simulink model "UNICO"  (R2023b)
settings: Solver=FixedStepDiscrete  StartTime=0.0  StopTime=inf  FixedStep=Control.DT  RelTol=1e-3
undefined symbols (not defined in the file): Control
libraries: cstblocks x5, simulink x2
(part 2 of 3)

== system UNICO/Echo print/Enabled Subsystem ==
  Init : Inport
  Params : Inport  Port=2
  KpAr : Inport  Port=3
  KiAr : Inport  Port=4
  KpBr : Inport  Port=5
  KiBr : Inport  Port=6
  Max_Rat : Inport  Port=7
  Params_WS_F : Inport  Port=8
  Enable : EnablePort
  Echo1 : MATLAB Function  TreatAsAtomicUnit=on
  wires:
  Init/1 -> Echo1/1(Init)
  Params_WS_F/1 -> Echo1/8(Params_WS_F)
  Max_Rat/1 -> Echo1/7(Max_Rat)
  KiAr/1 -> Echo1/4(KiAr)
  KpAr/1 -> Echo1/3(KpAr)
  Params/1 -> Echo1/2(Params)
  KpBr/1 -> Echo1/5(KpBr)
  KiBr/1 -> Echo1/6(KiBr)

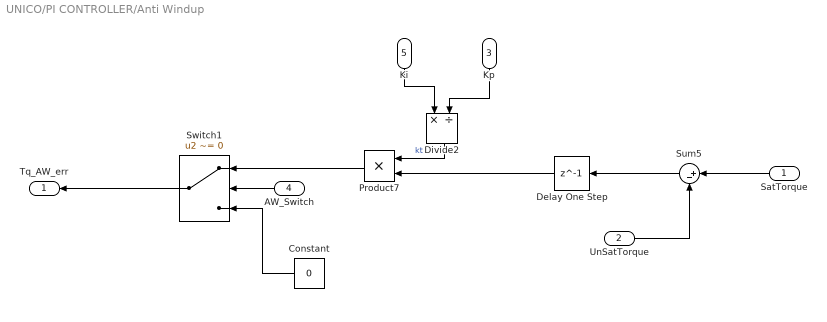
== system UNICO/PI CONTROLLER/Anti Windup ==
  SatTorque : Inport
  UnSatTorque : Inport  Port=2
  Kp : Inport  Port=3
  AW_Switch : Inport  Port=4
  Ki : Inport  Port=5
  Constant : Constant  Value=0
  Delay One Step : Delay  DelayLength=1
  Divide2 : Product  Inputs=*/
  Product7 : Product
  Sum5 : Sum  Inputs=|+-
  Switch1 : Switch  Criteria=u2 ~= 0  SaturateOnIntegerOverflow=off  InputSameDT=off
  Tq_AW_err : Outport
  wires:
  Sum5/1 -> Delay One Step/1
  Ki/1 -> Divide2/1
  SatTorque/1 -> Sum5/1
  Divide2/1 -> Product7/1  "kt"
  Delay One Step/1 -> Product7/2
  Kp/1 -> Divide2/2
  UnSatTorque/1 -> Sum5/2
  Product7/1 -> Switch1/1
  Switch1/1 -> Tq_AW_err/1
  Constant/1 -> Switch1/3
  AW_Switch/1 -> Switch1/2

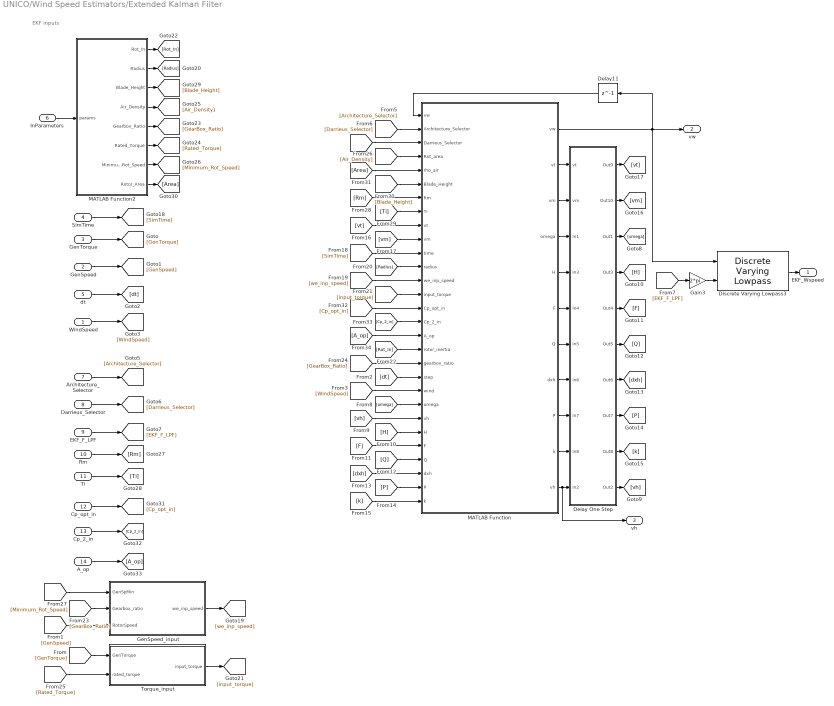
== system UNICO/Wind Speed Estimators/Extended Kalman Filter ==
  note: EKF inputs
  WindSpeed : Inport
  GenSpeed : Inport  Port=2
  GenTorque : Inport  Port=3
  SimTime : Inport  Port=4
  dt : Inport  Port=5
  InParameters : Inport  Port=6
  Architecture_Selector : Inport  Port=7
  Darrieus_Selector : Inport  Port=8
  EKF_F_LPF : Inport  Port=9
  Rm : Inport  Port=10
  Ti : Inport  Port=11
  Cp_opt_in : Inport  Port=12
  Cp_2_in : Inport  Port=13
  A_op : Inport  Port=14
  Delay One Step : Subsystem
  Delay11 : Delay  DelayLength=1
  Discrete Varying Lowpass3 : cstblocks/Linear Parameter Varying/Discrete Varying Lowpass  N=1  w0=0  Ts=Control.DT
  Gain3 : Gain  Gain=2*pi
  GenSpeed_input : MATLAB Function  TreatAsAtomicUnit=on
  MATLAB Function : MATLAB Function  TreatAsAtomicUnit=on
  MATLAB Function2 : MATLAB Function  TreatAsAtomicUnit=on
  Torque_input : MATLAB Function  TreatAsAtomicUnit=on
  EKF_Wspeed : Outport
  vw : Outport  Port=2
  vh : Outport  Port=3
  wires:
  [Radius] -> MATLAB Function/12(radius)
  [GearBox_Ratio] -> GenSpeed_input/2(Gearbox_ratio)
  [Minimum_Rot_Speed] -> GenSpeed_input/1(GenSpMin)
  [Rated_Torque] -> Torque_input/2(rated_torque)
  [Rot_In] -> MATLAB Function/18(rotor_inertia)
  Delay11/1 -> MATLAB Function/1("vw ")
  MATLAB Function/1(vw) -> vw/1, Delay11/1, Discrete Varying Lowpass3/1
  [EKF_F_LPF] -> Gain3/1
  Gain3/1 -> Discrete Varying Lowpass3/2
  Discrete Varying Lowpass3/1 -> EKF_Wspeed/1
  InParameters/1 -> MATLAB Function2/1(params)
  GenTorque/1 -> [GenTorque]
  [GenTorque] -> Torque_input/1(GenTorque)
  GenSpeed/1 -> [GenSpeed]
  [GenSpeed] -> GenSpeed_input/3(RotorSpeed)
  dt/1 -> [dt]
  [dt] -> MATLAB Function/20(step)
  WindSpeed/1 -> [WindSpeed]
  [WindSpeed] -> MATLAB Function/21(wind)
  Architecture_Selector/1 -> [Architecture_Selector]
  Darrieus_Selector/1 -> [Darrieus_Selector]
  EKF_F_LPF/1 -> [EKF_F_LPF]
  MATLAB Function/4(omega) -> Delay One Step/3(In1)
  MATLAB Function/5(H) -> Delay One Step/4(In3)
  MATLAB Function/6(F) -> Delay One Step/5(In4)
  MATLAB Function/7(Q) -> Delay One Step/6(In5)
  MATLAB Function/8(dxh) -> Delay One Step/7(In6)
  MATLAB Function/9(P) -> Delay One Step/8(In7)
  MATLAB Function/10(k) -> Delay One Step/9(In8)
  Delay One Step/3(Out1) -> [omega]
  Delay One Step/10(Out2) -> [vh]
  Delay One Step/4(Out3) -> [H]
  Delay One Step/5(Out4) -> [F]
  Delay One Step/6(Out5) -> [Q]
  Delay One Step/7(Out6) -> [dxh]
  Delay One Step/8(Out7) -> [P]
  Delay One Step/9(Out8) -> [k]
  [omega] -> MATLAB Function/22("omega ")
  [vh] -> MATLAB Function/23("vh ")
  [H] -> MATLAB Function/24("H ")
  [F] -> MATLAB Function/25("F ")
  [Q] -> MATLAB Function/26("Q ")
  [dxh] -> MATLAB Function/27("dxh ")
  [P] -> MATLAB Function/28("P ")
  [k] -> MATLAB Function/29("k ")
  MATLAB Function/3(vm) -> Delay One Step/2(vm)
  MATLAB Function/2(vt) -> Delay One Step/1(vt)
  Delay One Step/1(Out9) -> [vt]
  Delay One Step/2(Out10) -> [vm]
  [vt] -> MATLAB Function/9("vt ")
  [vm] -> MATLAB Function/10("vm ")
  SimTime/1 -> [SimTime]
  [SimTime] -> MATLAB Function/11(time)
  GenSpeed_input/1(we_inp_speed) -> [we_inp_speed]
  [we_inp_speed] -> MATLAB Function/13(we_inp_speed)
  MATLAB Function2/2(Radius) -> [Radius]
  Torque_input/1(input_torque) -> [input_torque]
  [input_torque] -> MATLAB Function/14(input_torque)
  MATLAB Function2/1(Rot_In) -> [Rot_In]
  MATLAB Function2/5(Gearbox_Ratio) -> [GearBox_Ratio]
  [GearBox_Ratio] -> MATLAB Function/19(gearbox_ratio)
  MATLAB Function2/6(Rated_Torque) -> [Rated_Torque]
  MATLAB Function2/4(Air_Density) -> [Air_Density]
  MATLAB Function2/7(Minimum_Rot_Speed) -> [Minimum_Rot_Speed]
  Rm/1 -> [Rm]
  Ti/1 -> [Ti]
  [Rm] -> MATLAB Function/7(Rm)
  [Ti] -> MATLAB Function/8(Ti)
  MATLAB Function2/3(Blade_Height) -> [Blade_Height]
  [Blade_Height] -> MATLAB Function/6(Blade_Height)
  [Air_Density] -> MATLAB Function/4(Rot_area)
  [Darrieus_Selector] -> MATLAB Function/3(Darrieus_Selector)
  [Architecture_Selector] -> MATLAB Function/2(Architecture_Selector)
  MATLAB Function2/8(Rotor_Area) -> [Area]
  [Area] -> MATLAB Function/5(rho_air)
  A_op/1 -> [A_op]
  Cp_2_in/1 -> [Cp_2_in]
  Cp_opt_in/1 -> [Cp_opt_in]
  [Cp_2_in] -> MATLAB Function/16(Cp_2_in)
  [Cp_opt_in] -> MATLAB Function/15(Cp_opt_in)
  [A_op] -> MATLAB Function/17(A_op)
  MATLAB Function/11(vh) -> vh/1, Delay One Step/10(In2)

== system UNICO/Wind Speed Estimators/Subsystem ==
  dt : Inport
  GenSpeed : Inport  Port=2
  Delay One Step : Delay  DelayLength=1
  Divide : Product  Inputs=*/
  Sum : Sum  Inputs=|+-
  GenAcc : Outport
  wires:
  GenSpeed/1 -> Sum/1, Delay One Step/1
  Delay One Step/1 -> Sum/2
  dt/1 -> Divide/2
  Sum/1 -> Divide/1
  Divide/1 -> GenAcc/1

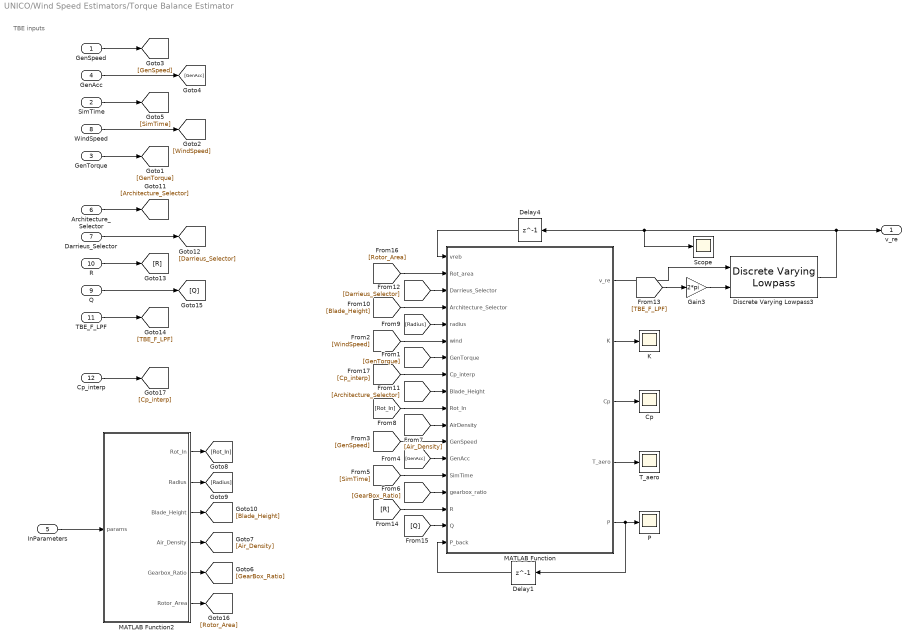
== system UNICO/Wind Speed Estimators/Torque Balance Estimator ==
  note: TBE inputs
  GenSpeed : Inport
  SimTime : Inport  Port=2
  GenTorque : Inport  Port=3
  GenAcc : Inport  Port=4
  InParameters : Inport  Port=5
  Architecture_Selector : Inport  Port=6
  Darrieus_Selector : Inport  Port=7
  WindSpeed : Inport  Port=8
  Q : Inport  Port=9
  R : Inport  Port=10
  TBE_F_LPF : Inport  Port=11
  Cp_interp : Inport  Port=12
  Cp : Scope
  Delay1 : Delay  DelayLength=1
  Delay4 : Delay  DelayLength=1
  Discrete Varying Lowpass3 : cstblocks/Linear Parameter Varying/Discrete Varying Lowpass  N=1  w0=0  Ts=Control.DT
  Gain3 : Gain  Gain=2*pi
  K : Scope
  MATLAB Function : MATLAB Function  TreatAsAtomicUnit=on
  MATLAB Function2 : MATLAB Function  TreatAsAtomicUnit=on
  P : Scope
  Scope : Scope
  T_aero : Scope
  v_re : Outport
  wires:
  Delay4/1 -> MATLAB Function/1(vreb)
  MATLAB Function/1(v_re) -> Discrete Varying Lowpass3/1
  [TBE_F_LPF] -> Gain3/1
  Gain3/1 -> Discrete Varying Lowpass3/2
  Discrete Varying Lowpass3/1 -> v_re/1, Delay4/1, Scope/1
  MATLAB Function/5(P) -> Delay1/1, P/1
  Delay1/1 -> MATLAB Function/18(P_back)
  MATLAB Function/2(K) -> K/1
  MATLAB Function/3(Cp) -> Cp/1
  MATLAB Function/4(T_aero) -> T_aero/1
  InParameters/1 -> MATLAB Function2/1(params)
  GenTorque/1 -> [GenTorque]
  [GenTorque] -> MATLAB Function/7(GenTorque)
  WindSpeed/1 -> [WindSpeed]
  [WindSpeed] -> MATLAB Function/6(wind)
  [GenSpeed] -> MATLAB Function/12(GenSpeed)
  GenSpeed/1 -> [GenSpeed]
  GenAcc/1 -> [GenAcc]
  [GenAcc] -> MATLAB Function/13(GenAcc)
  SimTime/1 -> [SimTime]
  [SimTime] -> MATLAB Function/14(SimTime)
  MATLAB Function2/5(Gearbox_Ratio) -> [GearBox_Ratio]
  [GearBox_Ratio] -> MATLAB Function/15(gearbox_ratio)
  [Air_Density] -> MATLAB Function/11(AirDensity)
  MATLAB Function2/4(Air_Density) -> [Air_Density]
  MATLAB Function2/1(Rot_In) -> [Rot_In]
  [Rot_In] -> MATLAB Function/10(Rot_In)
  MATLAB Function2/2(Radius) -> [Radius]
  MATLAB Function2/3(Blade_Height) -> [Blade_Height]
  [Blade_Height] -> MATLAB Function/4(Architecture_Selector)
  [Radius] -> MATLAB Function/5(radius)
  Architecture_Selector/1 -> [Architecture_Selector]
  [Architecture_Selector] -> MATLAB Function/9(Blade_Height)
  Darrieus_Selector/1 -> [Darrieus_Selector]
  [Darrieus_Selector] -> MATLAB Function/3(Darrieus_Selector)
  R/1 -> [R]
  Q/1 -> [Q]
  TBE_F_LPF/1 -> [TBE_F_LPF]
  [R] -> MATLAB Function/16(R)
  [Q] -> MATLAB Function/17(Q)
  MATLAB Function2/6(Rotor_Area) -> [Rotor_Area]
  [Rotor_Area] -> MATLAB Function/2(Rot_area)
  [Cp_interp] -> MATLAB Function/8(Cp_interp)
  Cp_interp/1 -> [Cp_interp]

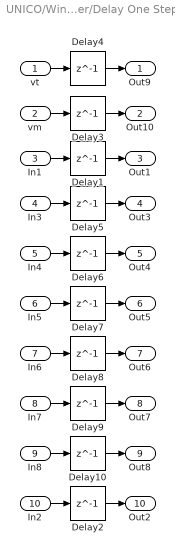
== system UNICO/Wind Speed Estimators/Extended Kalman Filter/Delay One Step ==
  vt : Inport
  vm : Inport  Port=2
  In1 : Inport  Port=3
  In3 : Inport  Port=4
  In4 : Inport  Port=5
  In5 : Inport  Port=6
  In6 : Inport  Port=7
  In7 : Inport  Port=8
  In8 : Inport  Port=9
  In2 : Inport  Port=10
  Delay{1..10} (10 alike) : Delay  DelayLength=1
  Out9 : Outport
  Out10 : Outport  Port=2
  Out1 : Outport  Port=3
  Out3 : Outport  Port=4
  Out4 : Outport  Port=5
  Out5 : Outport  Port=6
  Out6 : Outport  Port=7
  Out7 : Outport  Port=8
  Out8 : Outport  Port=9
  Out2 : Outport  Port=10
  wires:
  Delay8/1 -> Out6/1
  In7/1 -> Delay9/1
  Delay5/1 -> Out3/1
  Delay2/1 -> Out2/1
  In4/1 -> Delay6/1
  In1/1 -> Delay1/1
  In5/1 -> Delay7/1
  In6/1 -> Delay8/1
  In8/1 -> Delay10/1
  Delay9/1 -> Out7/1
  Delay6/1 -> Out4/1
  Delay7/1 -> Out5/1
  Delay10/1 -> Out8/1
  In2/1 -> Delay2/1
  In3/1 -> Delay5/1
  Delay1/1 -> Out1/1
  Delay4/1 -> Out9/1
  vt/1 -> Delay4/1
  vm/1 -> Delay3/1
  Delay3/1 -> Out10/1

== matlab function UNICO/PI CONTROLLER/Saturate  torque ==
  data: Unsat_Tq input; Gen_Tq output; Params input; time input
function Gen_Tq = fcn(Unsat_Tq, Params, time)


Min_Tq = Params(7);  %minimum torque value  [Nm]
Max_Tq = Params(8);  % maximum torque value  [Nm]

if time < -1   % at the beginning of the simulation do not apply torque saturation to avoid divergence
    Gen_Tq = Unsat_Tq;
else

    if Unsat_Tq > Max_Tq  % if torque from controller is larger than maximum saturation value
        

        Gen_Tq = Max_Tq;  % set the torque value to the MaxTq

    elseif Unsat_Tq < Min_Tq  % if torque from controller is smaller than minimum saturation value

        Gen_Tq = Min_Tq;  % set torque value to MinTq

    else   % if torque from controller is within the max and min values, do not modify the output torque value

        Gen_Tq = Unsat_Tq;


    end
end

== matlab function UNICO/Rate limiter ==
  data: Gen_Tq_b input; Gen_Tq input; s output; dMaxRate input; time input; dt input
function s = fcn(Gen_Tq_b,Gen_Tq,dMaxRate, time, dt)
% rate limiter applied only after *** seconds to allow for controller
% initialization
if time>0
    rate_lim_pos = dMaxRate; % rate limit for torque is simmetric
    rate_lim_neg = -dMaxRate;
    % calculate torque rate
    rate = (Gen_Tq-Gen_Tq_b)/dt;

    if rate > rate_lim_pos % if the torque rate is larger than the maximum allowed, set the torque using the maximum rate

        Gen_Tq = Gen_Tq_b+rate_lim_pos*dt;

    elseif rate < rate_lim_neg % if the torque rate is smaller than the minimum allowed, set the torque using the minimum rate

        Gen_Tq = Gen_Tq_b+rate_lim_neg*dt;

    end

else

end
% if the maximum torque rate is not violated
s = Gen_Tq;

== matlab function UNICO/MATLAB Function2 ==
  data: log1 input; y1 output; log2 input; log3 input; log4 input; y2 output; y3 output
function [y1, y2, y3] = log_to_file(log1, log2, log3, log4)
% log1      : [-]
% log2      : [-]
% log3      : [-]
% log4      : [-]

% y1, y2, y3 (pass-through)
y1 = log1;
y2 = log2;
y3 = log3;

persistent fid
if isempty(fid)
    % Corrected: used commas to separate arguments and removed extra semicolons
    fid = fopen('D:\Dario\Firenze_Maggio\Simulazioni_Sandia\UNICO_logger.txt', 'w');

    if fid == -1
        % Optional: use warning('Failed to open file'); to see if it fails in the console
        return;
    end

    % Standard header creation
    header = sprintf('log1[-]\tlog2[-]\tlog3[-]\tlog4[-]\n');
    fwrite(fid, header, 'char');
end

if fid ~= -1
    row = sprintf('%.6f\t%.6f\t%.6f\t%.6f\n', log1, log2, log3, log4);
    fwrite(fid, row, 'char');
end

== matlab function UNICO/Reference Speed Determination/WT_Controller ==
  data: WindSpeed input; GenSpeed input; GenSpeedRef output; Params input; Ref_Speed_F_Sw output; Ref_Speed_F_LPF output; Architecture_Selector input; Darrieus_Selector input
function [GenSpeedRef, Ref_Speed_F_Sw,Ref_Speed_F_LPF]  = WT_Controller(WindSpeed, GenSpeed, Params, Architecture_Selector, Darrieus_Selector)

% Load struct variables
R       = Params(1);                        % Rotor radius                                [m]
v_rt    = Params(2);                        % Rated wind speed                            [m/s]
Pt      = Params(4);                        % RatedPwr                                    [W]
w_rt    = Params(5);                        % RatedGenSpeed                               [rad/s]
eta     = Params(6);                        % Generator Efficiency                        [-]
w_min   = Params(9);                        % Minimum generator speed                     [rad/s]
r2      = Params(10);                       % Region 2 control mode                       [-]
TSR_opt = Params(15);                       % optimal TSR                                 [-]
Cpmaxval= Params(16);                       % max CP value                                [-]
r3      = Params(17);                       % Region 3 control mode                       [-]
m       = Params(18);                       % Angular coefficient Region 3 linear method  []
V_lin   = Params(19);                       % Wind speed to start linear reduction        [m/s]
TSR_R3 =  Params(26);                       % Region 3 Tip Speed Ratio                    [-]
Ref_Speed_F_Sw = Params(20);                % Reference speed filter switch               [-]
Ref_Speed_F_LPF = Params(21);               % Reference speed cut-off frequency           [Hz]
rho     = Params(22);                       % Air density                                 [kg/m^3]
Bld_Height = Params(24);                    %Blades Height (VAWT ONLY)                    [m]
Rot_area= Params(28);                       % Rotor Area (Eggbeater Type VAWT ONLY)       [m^2]

% Define parameters
v       = WindSpeed;                        % Reassign parameter
w_opt   = v*TSR_opt/R;                      % Optimum generator speed (corresponding to optimum TSR)
if Architecture_Selector == 2
    if Darrieus_Selector == 1
        A = Bld_Height*2*R;                 %Area for VAWT - H Type
    else
        A = Rot_area;                       %Area for VAWT - Eggbeater Type
    end
else
    A = pi*(R^2);                           %Area for HAWT
end

% Region 1 - Region 2 - Region 2 1/2
if v <= v_rt
    if r2 == 0
        w_ref = min(max(w_min,w_opt),w_rt);  
    else
        % for switching region
        if abs(w_rt-GenSpeed)<abs(w_min-GenSpeed)
            %region 2.5
            w_ref = w_rt;
        else
            % region 1.5
            w_ref = w_min;

        end

    end
       
% Region 3
else
    % Rated power tracking
    if r3 == 0
        Cp = Pt*eta/(0.5*rho*A*v^3);
        Cp    = min(max(0,Cp),Cpmaxval);
        TSR   = TSR_R3;
        w_ref = v*TSR/R;

    else %linear reduction 
        
        if v< V_lin
            w_ref = w_rt;
        else
            w_ref = w_rt+m*(v-V_lin);
            w_ref = max(w_ref,w_min);

        end
    end
end

GenSpeedRef = w_ref;  % PI controller reference rotational speed
end

== matlab function UNICO/Echo print/Enabled Subsystem/Echo1 ==
  data: Init input; Params input; KpAr input; KiAr input; KpBr input; KiBr input; Max_Rat input; Params_WS_F input
function fcn(Init, Params, KpAr, KiAr, KpBr, KiBr, Max_Rat, Params_WS_F)

R               = Params(1);  % Rotor radius [m]
v_rt            = Params(2);  % Rated wind speed  [m/s]
Rt_Tq           = Params(3);  % Rated torque  [Nm]
Pt              = Params(4);  % Rated Power [-]
w_rt            = Params(5);  % Rated Geerator Speed  [W]
eta             = Params(6);  % Generator Efficiency [-]
Min_Tq          = Params(7); % Minimum Torque [Nm]
Max_Tq          = Params(8);  % Maximum torque  [Nm]
w_min           = Params(9);  % Minimum generator speed  [rad/s]
r2              = Params(10);    % Region 2 control mode [-]
KSwitch         = Params(11);  % Switch for user defined k [-] 
Rgn2K           = Params(12);    %user defined K value [Nms^2/rad^2] 
SpdSwitch       = Params(13);  % velocity switch between Rgn 2 and 2 1/2 [rad/s]
w_minSwitch     = Params(14); % Velocity switch between Rgn 1.5 and 2 [rad/s]
TSR_opt         = Params(15);   %optimal TSR [-]
Cpmax           = Params(16);     % Optimal Cp [-]
r3              = Params(17);  % Region 3 control mode [-]
m               = Params(18);  % Angular coefficient Region 3 linear method
V_lin           = Params(19);  % Wind speed to start linear reduction [m/s]
Ref_Speed_F_Sw  = Params(20); % Reference speed filter switch [-]
Ref_Speed_F_LPF = Params(21); % Reference speed cut-off frequency [Hz]
rho             = Params(22);  % Air density             [kg/m^3]
Wind_Speed_F_Sw = Params_WS_F(1); % switch for wind speed Low-pass filter [-]
Wind_Speed_F_LPF= Params_WS_F(2); % wind speed low pass filter frequency [Hz]
Gen_Speed_F_Sw  = Params_WS_F(3); % Switch for generator speed low-pass filter [-]
Gen_Speed_F_LPF = Params_WS_F(4); % Generator speed low pass frequeny [Hz]




if Init == 0
    
f_echo = fopen('UNICO_echo.txt','w');
fprintf(f_echo,'UNICO CONTROLLER SIMULATION INPUT \n');
fprintf(f_echo,'Rotor radius [m]:                           %f \n',R);
fprintf(f_echo,'Rated wind speed [m/s]:                     %f \n',v_rt);
fprintf(f_echo,'Rated Torque [Nm]:                          %f \n',Rt_Tq);
fprintf(f_echo,'Rated power [W]:                            %f \n',Pt);
fprintf(f_echo,'Rated generator speed [rad/s]:              %f \n',w_rt);
fprintf(f_echo,'Generator efficiency [-]:                   %f \n',eta);
fprintf(f_echo,'Minimum Torque [Nm]:                        %f \n',Min_Tq);
fprintf(f_echo,'Maximum generator torque [Nm]:              %f \n',Max_Tq);
fprintf(f_echo,'Maximum generator torque rate [Nm/s]:       %f \n',Max_Rat);
fprintf(f_echo,'Minumum generator speed [rad/s]:            %f \n',w_min);
fprintf(f_echo, 'Region 2 control [-]:                      %f \n', r2);
fprintf(f_echo,'Switch for user defined K [-]:              %f \n',KSwitch);
fprintf(f_echo,'User defined K value [Nms^2/rad^2]:         %f \n',Rgn2K);
fprintf(f_echo,'Switch between Rgn2 and 2.5 [rad/s]:        %f \n',SpdSwitch);
fprintf(f_echo,'Switch between Rgn1.5 and 2 [rad/s]:        %f \n',w_minSwitch);
fprintf(f_echo,'Optimum TSR [-]:                            %f \n',TSR_opt);
fprintf(f_echo,'Maximum Cp value [-]:                       %f \n', Cpmax);
fprintf(f_echo,'Region 3 control [-]:                       %f \n',r3);
fprintf(f_echo,'Angular coefficient linear method []:       %f \n',m);
fprintf(f_echo,'Start reduction of ref velocity [m/s]:      %f \n', V_lin);
fprintf(f_echo,'Above rated PI Controller Kp [Nms/rad]:     %f \n',KpAr);
fprintf(f_echo,'Above rated PI Controller Ki [Nm/rad]:      %f \n',KiAr);
fprintf(f_echo,'Below rated PI Controller Kp [Nms/rad]:     %f \n',KpBr);
fprintf(f_echo,'Below rated PI Controller Ki [Nm/rad]:      %f \n',KiBr);
fprintf(f_echo,'Switch Wind speed filter [-]:               %f \n',Wind_Speed_F_Sw);
fprintf(f_echo,'Wind speed lowpass frequency[Hz]:           %f \n',Wind_Speed_F_LPF);
fprintf(f_echo,'Switch Generator speed filter [-]:          %f \n',Gen_Speed_F_Sw);
fprintf(f_echo,'Generator speed lowpass frequency [Hz]:     %f \n',Gen_Speed_F_LPF);
fprintf(f_echo,'Switch reference speed filter [-]:          %f \n',Ref_Speed_F_Sw);
fprintf(f_echo,'Reference speed lowpass frequency [Hz]:     %f \n',Ref_Speed_F_LPF);
fprintf(f_echo,'Air density [kg/m^3]:                       %f \n',rho);
fclose(f_echo);

end

== matlab function UNICO/Extract Signals & Filtering/MATLAB Function ==
  data: w0 input; freq input; Ts input; u input; y output
function y = discreteVaryingLowpass(w0, freq, Ts, u)
% DISCRETEVARYINGLOWPASS Implements a 1st-order variable Butterworth filter.
%
% INPUTS:
%   u    : Current input signal
%   freq : Cutoff frequency in rad/s (can vary at each step)
%   Ts   : Sample time in seconds
%   w0   : Pre-warping frequency (rad/s). Set to 0 for standard Tustin.
%
% OUTPUT:
%   y    : Filtered output signal

    % Persistent variables to maintain state between time steps
    persistent u_prev y_prev
    
    % Initialization on the first run
    if isempty(u_prev)
        u_prev = 0;
        y_prev = 0;
    end

    % --- 1. Pre-warping Gain (K) ---
    % Standard Bilinear (Tustin) transform uses K = 2/Ts.
    % If a pre-warping frequency w0 is provided, K is adjusted.
    if w0 <= 0
        K = 2 / Ts;
    else
        K = w0 / tan(w0 * Ts / 2);
    end

    % --- 2. Variable Coefficient Calculation ---
    % Continuous Transfer Function: H(s) = freq / (s + freq)
    % Substitution: s = K * (z-1) / (z+1)
    
    denominator = (K + freq);
    b0 = freq / denominator;
    b1 = b0;                     % For 1st order Tustin, b0 always equals b1
    a1 = (freq - K) / denominator;

    % --- 3. Difference Equation ---
    % Standard Direct Form I implementation:
    % y[n] = b0*u[n] + b1*u[n-1] - a1*y[n-1]
    y = b0*u + b1*u_prev - a1*y_prev;

    % --- 4. State Update ---
    u_prev = u;
    y_prev = y;
end

== matlab function UNICO/Pitch Controller/Saturate  pitch ==
  data: pitch_max input; u input; y output; pitch_min input
function y = fcn(pitch_max, u, pitch_min)

lim_sup = pitch_max;    % Maximum blade pitch angle value [rad]

lim_inf = pitch_min;    % Minimum blade pitch angle value [rad]

if u > lim_sup          % If balde pitch angle from controller is larger than maximum saturation value

    y = lim_sup;        % Set blade pitch angle value to the lim_sup

elseif u < lim_inf      % If blade picth angle from controller is smaller than minimum saturation value

    y = lim_inf;        % Set blade picth angle value to the lim_inf

else                    % If blade picth angle from controller is within the max and min values, do not modify the output blade picth angle value

    y = u;      

end

end

== matlab function UNICO/Notch Filter/MATLAB Function ==
  data: DesGenSpeed input; BladePassFreq output; InPar input
function BladePassFreq = calculateBladePassFreq(DesGenSpeed, InPar)

    N_blades = InPar(23);

    % Converts rad/s of the generator to Hz of blade passage
    BladePassFreq = (N_blades * DesGenSpeed) / (2 * pi);
    
end

== matlab function UNICO/Extract Signals & Filtering/MATLAB Function1 ==
  data: w0 input; freq input; Ts input; u input; y output
function y = discreteVaryingLowpass(w0, freq, Ts, u)
% DISCRETEVARYINGLOWPASS Implements a 1st-order variable Butterworth filter.
%
% INPUTS:
%   u    : Current input signal
%   freq : Cutoff frequency in rad/s (can vary at each step)
%   Ts   : Sample time in seconds
%   w0   : Pre-warping frequency (rad/s). Set to 0 for standard Tustin.
%
% OUTPUT:
%   y    : Filtered output signal

    % Persistent variables to maintain state between time steps
    persistent u_prev y_prev
    
    % Initialization on the first run
    if isempty(u_prev)
        u_prev = 0;
        y_prev = 0;
    end

    % --- 1. Pre-warping Gain (K) ---
    % Standard Bilinear (Tustin) transform uses K = 2/Ts.
    % If a pre-warping frequency w0 is provided, K is adjusted.
    if w0 <= 0
        K = 2 / Ts;
    else
        K = w0 / tan(w0 * Ts / 2);
    end

    % --- 2. Variable Coefficient Calculation ---
    % Continuous Transfer Function: H(s) = freq / (s + freq)
    % Substitution: s = K * (z-1) / (z+1)
    
    denominator = (K + freq);
    b0 = freq / denominator;
    b1 = b0;                     % For 1st order Tustin, b0 always equals b1
    a1 = (freq - K) / denominator;

    % --- 3. Difference Equation ---
    % Standard Direct Form I implementation:
    % y[n] = b0*u[n] + b1*u[n-1] - a1*y[n-1]
    y = b0*u + b1*u_prev - a1*y_prev;

    % --- 4. State Update ---
    u_prev = u;
    y_prev = y;
end

== matlab function UNICO/Region Switch  ==
  data: WindSpeed input; GenSpeed input; PI_GenTq input; Architecture_Selector input; Darrieus_Selector input; GenTq output; Params input
function GenTq = Rgn2_Fcn(WindSpeed, GenSpeed, PI_GenTq, Architecture_Selector, Darrieus_Selector, Params)

% Load R struct variables
R       = Params(1);                        % Rotor radius                              [m]
v_rt    = Params(2);                        % Rated power wind speed                    [m/s]
w_rt    = Params(5);                        % Rated generator speed                     [rad/s]
w_min   = Params(9);                        % Minimum generator speed                   [rad/s]
r2      = Params(10);                       % Region 2 control mode  {0: optimum tsr tracking; 1: kw^2 torque law}
KSwitch = Params(11);                       % switch for user defined k
Rgn2K = Params(12);                         % user defined k {used only if KSwitch = 1}
SpdSwitch = Params(13);                     % speed switch from region 2 to 2 2 1/2     [rad/s]
w_minSwitch = Params(14);                   % Switch between region 1.5 and 2           [rad/s]
TSR_opt = Params(15);                       % Optimum TSR                               [-]
Cpmax = Params(16);                         % max cp value                              [-]
rho     = Params(22);                       % Air density                               [kg/m^3]
Bld_Height = Params(24);                    % Blades Height (VAWT ONLY)                 [m]            
Rot_area = Params(28);                      %Rotor Area (VAWT - Eggbeater Type ONLY)    [m^2]

% Define parameters
wg  = GenSpeed;
v   = WindSpeed;
if KSwitch == 1
    K = Rgn2K;
else
    if Architecture_Selector == 1
        K   = 0.5*rho*pi*R^5*Cpmax/TSR_opt^3;  % K coefficient for HAWT
    else
        if Darrieus_Selector == 1
             K   = rho*R^4*Bld_Height*Cpmax/TSR_opt^3;  % K coefficient for VAWT - H Type
        else
             K = 0.5*rho*Rot_area*R^3*Cpmax/TSR_opt^3;  % K coefficient for VAWT - Eggbeater Type
        end
    end
end
w1  = SpdSwitch;            % switching rotational speed for region 2.5 to 3
Tg1 = K*w1^2;               % torque value at the switching rotational speed
w2 = w_minSwitch;           % switching rotational speed for region 1.5 to 2
Tg2 = K*(w2)^2;             % generator torque at the switching rotational speed from k-w^2 law
Tgmin = K*w_min^2;          % generator torque at minimum rotational speed from k-w^2 law

% kw^2 control mode
if r2 == 1

    % if we are in region 1.5 or 2
    if (wg < w1) && (v <= v_rt)
        % use k-w^2 law
        GenTq =  K*wg^2;
        if wg < w2 % if the generator speed is smaller than the 1.5 switching value
            if PI_GenTq < Tg2 && PI_GenTq > Tgmin

                % use linear interpolation to smooth the switch between the two
                % regions
                GenTq = Tg2+(PI_GenTq-Tg2)/(w_min-w2)*(wg-w2);
               
            elseif PI_GenTq < Tgmin

                % in region 1.5 use TSR tracking to track the minimum speed
                % defined by the user
                GenTq = PI_GenTq;
                
            end
        end

    elseif (wg < w_rt) && (v <= v_rt)
        % region 2.5, smoothing of switch between region 2 and 3
        GenTq = Tg1+(PI_GenTq-Tg1)/(w_rt-w1)*(wg-w1);
    else
        % region 3
        GenTq = PI_GenTq;
    end
    % tsr tracking control mode
else
    GenTq = PI_GenTq;
end

== matlab function UNICO/Set Point Smoother/Rated_Power ==
  data: params input; y output
function y = fcn(params)
% extracting Turbine rated power from In_Parameters vector
y = params(4);  % Rated Power [W]

end

== matlab function UNICO/Set Point Smoother/MATLAB Function ==
  data: params input; w_rt output
function w_rt = fcn(params)
% extracting the reference generator speed  
w_rt = params(5);  

end

== matlab function UNICO/Extract Signals & Filtering/MATLAB Function2 ==
  data: w0 input; freq input; Ts input; u input; y output
function y = discreteVaryingLowpass(w0, freq, Ts, u)
% DISCRETEVARYINGLOWPASS Implements a 1st-order variable Butterworth filter.
%
% INPUTS:
%   u    : Current input signal
%   freq : Cutoff frequency in rad/s (can vary at each step)
%   Ts   : Sample time in seconds
%   w0   : Pre-warping frequency (rad/s). Set to 0 for standard Tustin.
%
% OUTPUT:
%   y    : Filtered output signal

    % Persistent variables to maintain state between time steps
    persistent u_prev y_prev
    
    % Initialization on the first run
    if isempty(u_prev)
        u_prev = 0;
        y_prev = 0;
    end

    % --- 1. Pre-warping Gain (K) ---
    % Standard Bilinear (Tustin) transform uses K = 2/Ts.
    % If a pre-warping frequency w0 is provided, K is adjusted.
    if w0 <= 0
        K = 2 / Ts;
    else
        K = w0 / tan(w0 * Ts / 2);
    end

    % --- 2. Variable Coefficient Calculation ---
    % Continuous Transfer Function: H(s) = freq / (s + freq)
    % Substitution: s = K * (z-1) / (z+1)
    
    denominator = (K + freq);
    b0 = freq / denominator;
    b1 = b0;                     % For 1st order Tustin, b0 always equals b1
    a1 = (freq - K) / denominator;

    % --- 3. Difference Equation ---
    % Standard Direct Form I implementation:
    % y[n] = b0*u[n] + b1*u[n-1] - a1*y[n-1]
    y = b0*u + b1*u_prev - a1*y_prev;

    % --- 4. State Update ---
    u_prev = u;
    y_prev = y;
end

== matlab function UNICO/Wind Speed Estimators/Torque Balance Estimator/MATLAB Function ==
  data: vreb input; Rot_area input; Darrieus_Selector input; Architecture_Selector input; radius input; wind input; GenTorque input; Cp_interp input; Blade_Height input; v_re output; K output; Cp output; T_aero output; Rot_In input; AirDensity input; GenSpeed input; GenAcc input; SimTime input; gearbox_ratio input; R input; Q input; P_back input; P output
function [v_re,K,Cp,T_aero,P] = fcn(vreb,Rot_area, Darrieus_Selector, Architecture_Selector, radius,wind,GenTorque,Cp_interp, Blade_Height, Rot_In,AirDensity,GenSpeed,GenAcc,SimTime,gearbox_ratio,R, Q, P_back)
if Architecture_Selector == 2
    if Darrieus_Selector == 1
        A = Blade_Height*2*radius; % Area VAWT - H Type
    else
        A = Rot_area; % Area VAWT - Eggbeater Type
    end
else
    A=pi*(radius)^2; % Area HAWT
end

% Initialization
if SimTime < 6 % If time is less than 6 seconds, set initial values
    v_re=wind;    % Set estimated wind speed equal to actual wind speed
    P=1;          % Initialize state estimation error covariance
    K=0;          % Initialize Kalman gain factor
    Cp=0;         % Initialize power coefficient
    T_aero=0;     % Initialize aerodynamic torque
else
    Cp=Cp_interp;                                           % Cp already interpolated in C
    Tfriction=0.04*GenTorque;                               % Calculate friction torque
    Trotor=Rot_In*GenAcc;                                   % Calculate rotor torque from inertia
    T_aero=Trotor+GenTorque*gearbox_ratio+Tfriction;        % Compute aerodynamic torque from torque balance
    vre_cub=T_aero*2*GenSpeed/(AirDensity*A*Cp);            % Compute the cube of the estimated effective wind speed
    vre=nthroot(vre_cub,3);                                 % Compute the effective wind speed
    P_pred=P_back+Q;                                        % Compute state estimation error covariance from the previous step
    y=vre-vreb;                                             % Compute the wind speed difference between the predicted and the value from the previous step
    K=P_pred/(P_pred+R);                                    % Compute Kalman gain factor
    v_re=vreb+K*y;                                          % Update estimated wind speed
    P=(1-K)*P_pred;                                         % Update state estimation error covariance
end
end

== matlab function UNICO/Extract Signals & Filtering/MATLAB Function3 ==
  data: w0 input; freq input; Ts input; u input; y output
function y = discreteVaryingLowpass(w0, freq, Ts, u)
% DISCRETEVARYINGLOWPASS Implements a 1st-order variable Butterworth filter.
%
% INPUTS:
%   u    : Current input signal
%   freq : Cutoff frequency in rad/s (can vary at each step)
%   Ts   : Sample time in seconds
%   w0   : Pre-warping frequency (rad/s). Set to 0 for standard Tustin.
%
% OUTPUT:
%   y    : Filtered output signal

    % Persistent variables to maintain state between time steps
    persistent u_prev y_prev
    
    % Initialization on the first run
    if isempty(u_prev)
        u_prev = 0;
        y_prev = 0;
    end

    % --- 1. Pre-warping Gain (K) ---
    % Standard Bilinear (Tustin) transform uses K = 2/Ts.
    % If a pre-warping frequency w0 is provided, K is adjusted.
    if w0 <= 0
        K = 2 / Ts;
    else
        K = w0 / tan(w0 * Ts / 2);
    end

    % --- 2. Variable Coefficient Calculation ---
    % Continuous Transfer Function: H(s) = freq / (s + freq)
    % Substitution: s = K * (z-1) / (z+1)
    
    denominator = (K + freq);
    b0 = freq / denominator;
    b1 = b0;                     % For 1st order Tustin, b0 always equals b1
    a1 = (freq - K) / denominator;

    % --- 3. Difference Equation ---
    % Standard Direct Form I implementation:
    % y[n] = b0*u[n] + b1*u[n-1] - a1*y[n-1]
    y = b0*u + b1*u_prev - a1*y_prev;

    % --- 4. State Update ---
    u_prev = u;
    y_prev = y;
end

== matlab function UNICO/Extract Signals & Filtering/MATLAB Function4 ==
  data: w0 input; freq input; Ts input; u input; y output
function y = discreteVaryingLowpass(w0, freq, Ts, u)
% DISCRETEVARYINGLOWPASS Implements a 1st-order variable Butterworth filter.
%
% INPUTS:
%   u    : Current input signal
%   freq : Cutoff frequency in rad/s (can vary at each step)
%   Ts   : Sample time in seconds
%   w0   : Pre-warping frequency (rad/s). Set to 0 for standard Tustin.
%
% OUTPUT:
%   y    : Filtered output signal

    % Persistent variables to maintain state between time steps
    persistent u_prev y_prev
    
    % Initialization on the first run
    if isempty(u_prev)
        u_prev = 0;
        y_prev = 0;
    end

    % --- 1. Pre-warping Gain (K) ---
    % Standard Bilinear (Tustin) transform uses K = 2/Ts.
    % If a pre-warping frequency w0 is provided, K is adjusted.
    if w0 <= 0
        K = 2 / Ts;
    else
        K = w0 / tan(w0 * Ts / 2);
    end

    % --- 2. Variable Coefficient Calculation ---
    % Continuous Transfer Function: H(s) = freq / (s + freq)
    % Substitution: s = K * (z-1) / (z+1)
    
    denominator = (K + freq);
    b0 = freq / denominator;
    b1 = b0;                     % For 1st order Tustin, b0 always equals b1
    a1 = (freq - K) / denominator;

    % --- 3. Difference Equation ---
    % Standard Direct Form I implementation:
    % y[n] = b0*u[n] + b1*u[n-1] - a1*y[n-1]
    y = b0*u + b1*u_prev - a1*y_prev;

    % --- 4. State Update ---
    u_prev = u;
    y_prev = y;
end

== matlab function UNICO/Wind Speed Estimators/Extended Kalman Filter/MATLAB Function ==
  data: vw input; Architecture_Selector input; Darrieus_Selector input; Rot_area input; rho_air input; Blade_Height input; Rm input; Ti input; vw output; vt input; vm input; time input; vt output; radius input; we_inp_speed input; input_torque input; vm output; omega output; H output size=[1 3]; F output size=[3 3]; Q output size=[3 3]; dxh output size=[3 1]; P output size=[3 3]; k output size=[3 1]; vh output; Cp_opt_in input; Cp_2_in input; A_op input; rotor_inertia input; gearbox_ratio input; step input; wind input; omega input; vh input; H input size=[1 3]; F input size=[3 3]; Q input size=[3 3]; dxh input size=[3 1]; P input size=[3 3]; k input size=[3 1]
function [vw,vt,vm,omega,H,F,Q,dxh,P,k,vh] = fcn(vw,Architecture_Selector, Darrieus_Selector, Rot_area, rho_air, Blade_Height, Rm, Ti, vt,vm,time,radius,we_inp_speed,input_torque,Cp_opt_in,Cp_2_in,A_op,rotor_inertia,gearbox_ratio,step,wind,omega,vh,H,F,Q,dxh,P,k)
L=6*radius; % Define the turbulence length scale
I=eye(3);
% Initialization
if time < 10
    omega=we_inp_speed;             % Set initial rotor speed
    vt=0;                           % Initialize turbulence-induced wind speed
    vm=wind;                        % Set initial mean wind speed
    vh=wind;                        % Set initial hub-height wind speed
    H=[1,0,0];                      % Measurement matrix
    F=zeros(3,3);                   % Initialize system dynamics matrix
    Q=zeros(3,3);                   % Initialize process noise covariance matrix
    dxh=zeros(3,1);                 % Initialize state derivative vector
    P=[0.01,0,0;0,0.01,0;0,0,1];    % Initialize state covariance matrix
    k=zeros(3,1);                   % Initialize Kalman gain
    vw=vt+vm;                       % Compute total wind speed
% Extended Kalman Filter (EKF) based on Abbas' approach
else
    % Update state vector with current values
    xh=[omega;vt;vm];
    dt=step;            % Time step size

    if Architecture_Selector == 2
        if Darrieus_Selector == 1
            Area = Blade_Height*2*radius;
        else
            Area = Rot_area;
        end
    else
        Area=pi*(radius^2);           % Rotor swept area
    end

    % Cp_opt and Cp_2 already interpolated in C using vh and vw
    Cp_opt = Cp_opt_in;
    Cp_2 = Cp_2_in;

    % Define system dynamics matrix F (A_op already interpolated in C)
    F(1,1)=A_op;
    F(1,2)=rho_air*Area*3*Cp_opt*(vh^2)/(omega*2*rotor_inertia);
    F(1,3)=F(1,2);
    F(2,2)=-pi*vm/(2*L);
    F(2,3)=-pi*vt/(2*L);

    % Define process noise covariance matrix Q
    Q(1,1)=0.00001;
    Q(2,2)=pi*(vm^3)*(Ti^2)/L;
    Q(3,3)=4/600;

    % Compute additional system parameters
    a=pi*vm/(2*L);

    % Compute aerodynamic torque
    tau=0.5*rho_air*Area*(vw^3)*Cp_2/we_inp_speed;

    % Compute state derivatives
    dxh(1,1)=(tau-gearbox_ratio*input_torque)/rotor_inertia;
    dxh(2,1)=-a*vt;
    dxh(3,1)=0;

    % Update state vector
    xh=xh+dxh*dt;

    % Update state covariance matrix
    P=P+dt*(F*P+P*F'+Q-k*Rm*k');

    % Compute Kalman gain
    S=(H*(P*H'))+Rm;
    k=P*H'/S;

    % Correct state estimate using Kalman filter
    xh=xh+k*(we_inp_speed-omega);
    P=(I-k*H)*P;

    % Extract updated state values
    omega=xh(1,1);      % Rotor speed
    vt=xh(2,1);         % Turbulence-induced wind speed
    vm=xh(3,1);         % Mean wind speed
    vh=vt+vm;           % Hub-height wind speed
    vw=vm+vt;           % Estimated (total) wind speed
end
end

== matlab function UNICO/Set Point Smoother/Gen_Ref_Pitch ==
  data: params input; delta_omega input; y output
function y = fcn(params, delta_omega)
% defining the new generator speed reference for the pitch controller
w_rt = params(5);  %Rated Generetor Speed as a Reference for pitch Control [rad/s]
 
if delta_omega < 0                  % In Region 2.5 modify the reference generator speed to avoid conflict with pitch controller

    y = w_rt - delta_omega;         % Following Abbas's rules

else                                % In Region 3 do no modify the reference generator speed

    y = w_rt;

end

end

== matlab function UNICO/Wind Speed Estimators/Extended Kalman Filter/GenSpeed_input ==
  data: GenSpMin input; we_inp_speed output; Gearbox_ratio input; RotorSpeed input
function we_inp_speed = fcn(GenSpMin,Gearbox_ratio,RotorSpeed)
% Function to ensure the rotor speed does not fall below a minimum threshold

if RotorSpeed < 0.25*GenSpMin/Gearbox_ratio         % Check if the rotor speed is below 25% of the minimum generator speed, adjusted by the gearbox ratio
    
    we_inp_speed = 0.25*GenSpMin/Gearbox_ratio;     % Set the input speed to the minimum allowable value

else                                                % Otherwise, use the actual rotor speed

    we_inp_speed = RotorSpeed;

end

end

== matlab function UNICO/Pitch Rate Limiter/Rate limiter ==
  data: u_b input; u input; s output; Pitch_Rate input; dt input
function s = fcn(u_b,u,Pitch_Rate, dt)

rate_lim_pos = Pitch_Rate; % rate limit for pitch is simmetric
rate_lim_neg = -Pitch_Rate;

% calculate pitch rate
rate = (u-u_b)/dt;

if rate > rate_lim_pos % if the pitch rate is larger than the maximum allowed, set the pitch using the maximum rate

    s = u_b+rate_lim_pos*dt;

elseif rate < rate_lim_neg % if the pitch rate is smaller than the minimum allowed, set the pitch using the minimum rate

    s = u_b+rate_lim_neg*dt;

else

    s = u;  % if the maximum pitch rate is not violated

end

== matlab function UNICO/Wind Speed Estimators/Extended Kalman Filter/Torque_input ==
  data: GenTorque input; input_torque output; rated_torque input
function input_torque = fcn(GenTorque,rated_torque)
% Function to limit the generator torque to a minimum threshold

if GenTorque < 0.001*rated_torque               % If the generator torque is below 0.001 times the rated torque
    
    input_torque = 0.001*rated_torque;          % Set the input torque to the minimum allowable value

else                                            % Otherwise, use the actual generator torque

    input_torque = GenTorque;

end

end

== matlab function UNICO/Wind Speed Estimators/MATLAB Function ==
  data: WSE_Mode input; TBE_WSpeed input; Raw_WSpeed input; WSpeed output; EKF_WSpeed input
function WSpeed = fcn(WSE_Mode, TBE_WSpeed, Raw_WSpeed, EKF_WSpeed)
if WSE_Mode == 1
    WSpeed = TBE_WSpeed;
elseif WSE_Mode == 2
    WSpeed = EKF_WSpeed;
else
    WSpeed = Raw_WSpeed;
end

== matlab function UNICO/Set Point Smoother/GenSpeed_Ref_Torque_Controller ==
  data: Gen_Ref_torq input; delta_omega input; y output
function y = fcn(Gen_Ref_torq, delta_omega)
% Defining the new generator speed reference for the torque controller

if delta_omega >= 0                     % In Region 2.5 and 3 modify the reference generator speed to avoid conflict with pitch controller

    y = Gen_Ref_torq - delta_omega;     % Following Abbas's rules

else                                    % In Region 2 do no modify the reference generator speed

    y = Gen_Ref_torq;                   

end

end

== matlab function UNICO/Wind Speed Estimators/Extended Kalman Filter/MATLAB Function2 ==
  data: params input; Rot_In output; Radius output; Blade_Height output; Air_Density output; Gearbox_Ratio output; Rated_Torque output; Minimum_Rot_Speed output; Rotor_Area output
function [Rot_In, Radius, Blade_Height, Air_Density, Gearbox_Ratio, Rated_Torque, Minimum_Rot_Speed, Rotor_Area] = fcn(params)
% extracting the generator speed reference   
Radius = params(1); 
Air_Density = params(22);
Blade_Height = params(24);
Rot_In = params(25);
Gearbox_Ratio = params(27);
Rotor_Area = params(28);
Rated_Torque = params(3);
Minimum_Rot_Speed = params(9);
end

== matlab function UNICO/Extract Signals & Filtering/Filtering Block  ==
  data: windNF input; wnd output; wind input; GenSpeedNF input; GenSpeed input; Pitch input; PitchNF input; Tq input; TqNF input; Pwr input; PwrNF input; time input; omega output; ptch output; torque output; Power output; LPF_Starting_Time input
function [wnd,omega,ptch,torque,Power] = fcn(windNF, wind,GenSpeedNF, GenSpeed, Pitch, PitchNF, Tq, TqNF, Pwr, PwrNF, time, LPF_Starting_Time)

% At the beginning of the simulation do not apply filtering to avoid divergence

if time > LPF_Starting_Time

    wnd=wind;        % Wind speed filtered

    omega=GenSpeed;  % Generator speed filtered

    ptch=Pitch;      % Blade picth angle filtered

    torque=Tq;       % Generator torque filtered

    Power=Pwr;       % Generator power filtered

else

    wnd=windNF;         % Wind speed unfiltered

    omega=GenSpeedNF;   % Generator speed unfiltered

    ptch=PitchNF;       % Blade picth angle unfiltered

    torque=TqNF;        % Generator torque unfiltered

    Power=PwrNF;        % Generator power unfiltered

end

== matlab function UNICO/Wind Speed Estimators/Torque Balance Estimator/MATLAB Function2 ==
  data: params input; Rot_In output; Radius output; Blade_Height output; Air_Density output; Gearbox_Ratio output; Rotor_Area output
function [Rot_In, Radius, Blade_Height, Air_Density, Gearbox_Ratio, Rotor_Area]    = fcn(params)
% extracting the generator speed reference 
Radius = params(1); 
Rot_In = params(25);
Blade_Height = params(24);
Air_Density = params(22);
Gearbox_Ratio = params(27);
Rotor_Area = params(28);

end

== matlab function UNICO/Notch Filter/MATLAB Function2 ==
  data: SimTime input; GenSpeedUnfiltered input; GenSpeedFiltered input; Genspeed output
function Genspeed = fcn(SimTime, GenSpeedUnfiltered, GenSpeedFiltered)
Transient = 0;
if SimTime > Transient
Genspeed = GenSpeedFiltered ;
else 
Genspeed =  GenSpeedUnfiltered;
end

== matlab function UNICO/Notch Filter/MATLAB Function3 ==
  data: u input; Ts input; f0 input; Filt_GenTq output; zeta_z input; zeta_p input
function Filt_GenTq = notch_filter(u, Ts, f0, zeta_z, zeta_p)

persistent x1 x2 y1 y2 last_f0 last_Ts last_zz last_zp ...
           b0 b1 b2 a1 a2

% Initialize on first run
if isempty(x1)
    x1 = 0; x2 = 0;
    y1 = 0; y2 = 0;

    last_f0 = -1;
    last_Ts = -1;
    last_zz = -1;
    last_zp = -1;

    b0 = 1; b1 = 0; b2 = 0;
    a1 = 0; a2 = 0;
end

% Recompute coefficients only when parameters change AND Ts > 0
if (f0 ~= last_f0) || (Ts ~= last_Ts) || ...
   (zeta_z ~= last_zz) || (zeta_p ~= last_zp)

    if Ts > 0
        omega0 = 2*pi*f0;
        K  = 2 / Ts;
        K2 = K * K;
        w2 = omega0 * omega0;

        % Bilinear (Tustin) transform — numerator
        bz0 = K2 + 2*zeta_z*omega0*K + w2;
        bz1 = 2*w2 - 2*K2;
        bz2 = K2 - 2*zeta_z*omega0*K + w2;

        % Bilinear (Tustin) transform — denominator
        az0 = K2 + 2*zeta_p*omega0*K + w2;
        az1 = 2*w2 - 2*K2;
        az2 = K2 - 2*zeta_p*omega0*K + w2;

        % Normalize so a[0] = 1
        b0 = bz0 / az0;
        b1 = bz1 / az0;
        b2 = bz2 / az0;
        a1 = az1 / az0;
        a2 = az2 / az0;
    end
    % Always cache the current parameters (even when Ts=0)
    % so the next call (Ts=dt>0) recomputes correctly
    last_f0 = f0;
    last_Ts = Ts;
    last_zz = zeta_z;
    last_zp = zeta_p;
end

% IIR difference equation
Filt_GenTq = b0*u + b1*x1 + b2*x2 - a1*y1 - a2*y2;

% Update delay states
x2 = x1;
x1 = u;
y2 = y1;
y1 = Filt_GenTq;

end

== matlab function UNICO/PI CONTROLLER/Gain scheduling ==
  data: GenSpeed input; WindSpeed input; kp_ar input; Ki output; ki_ar input; kp_br input; ki_br input; Kp output; Params input
function [Ki,Kp] = fcn(GenSpeed, WindSpeed, kp_ar, ki_ar,kp_br, ki_br, Params)

R       = Params(1);  % Rotor radius           [m]
v_rt    = Params(2);  % Rated power wind speed [m/s]
w_rt    = Params(5);  % Rated generator speed  [rad/s]
r2      = Params(10);  % Region 2 control mode  {0: optimum tsr tracking; 1: kw^2 torque law}
SpdSwitch = Params(13); %generator speed for switch between region 2 and 2 1/2

% if we use TSR tracking in below rated conditions, schedule the PI
% coefficients
if r2 == 0

    if WindSpeed < v_rt && GenSpeed < w_rt

        % if GenSpeed <=SpdSwitch
        if GenSpeed <= SpdSwitch
            Kp = kp_br;
            Ki = ki_br;

        elseif GenSpeed > SpdSwitch && GenSpeed <w_rt
            % else

            Kp = kp_br+(kp_ar-kp_br)/(w_rt-SpdSwitch)*(GenSpeed-SpdSwitch);
            Ki = ki_br+(ki_ar-ki_br)/(w_rt-SpdSwitch)*(GenSpeed-SpdSwitch);

        else

            Kp = kp_ar;
            Ki = ki_ar;
            % end
        end


    else

        Kp = kp_ar;
        Ki = ki_ar;
    end

else
    % if k-w is used only a set of kp and ki is used
    Kp = kp_ar;
    Ki = ki_ar;

end

== matlab function UNICO/MATLAB Function1 ==
  data: dFPitch input; Pitch_Controller_Out input; Pitch_out output
function Pitch_out = Pitch_Switch(dFPitch, Pitch_Controller_Out)

if dFPitch <= -99
    Pitch_out = Pitch_Controller_Out;
else
    Pitch_out = dFPitch;
end

end
